simulink model "пример"  (R2023a)
settings: Solver=VariableStepAuto  StartTime=0.0  StopTime=10.0  RelTol=1e-3
libraries: simulink x1
settings Model: Creator=artemii  LastModifiedBy=Theomur

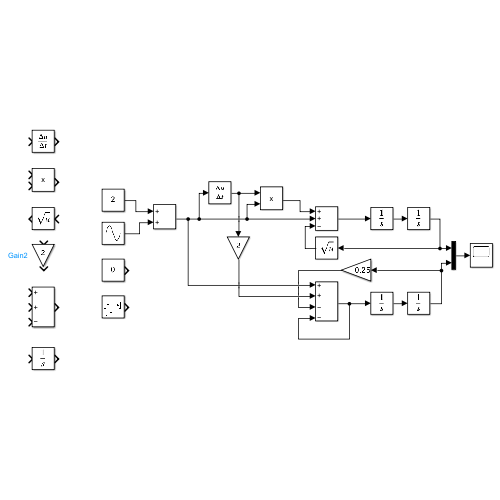
[thumbnail: Simulink's stored preview of the top-level diagram]
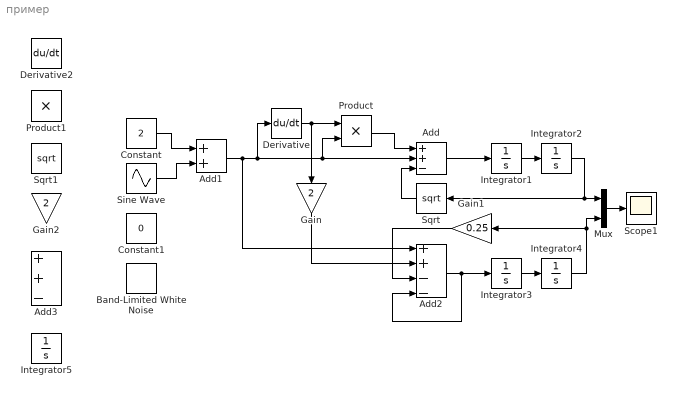
== system пример ==
  Add : Sum  Inputs=++-
  Add1 : Sum
  Add2 : Sum  Inputs=++--
  Add3 : Sum  Inputs=++-
  Band-Limited White Noise : simulink/Sources/Band-Limited White Noise  Cov=[0.1]  Ts=0.1  seed=[12345]
  Constant : Constant  Value=2
  Constant1 : Constant  Value=0
  Derivative : Derivative
  Derivative2 : Derivative
  Gain : Gain  Gain=2
  Gain1 : Gain  Gain=0.25
  Gain2 : Gain  Gain=2
  Integrator{1..5} (5 alike) : Integrator
  Mux : Mux  Inputs=2
  Product : Product
  Product1 : Product
  Scope1 : Scope
  Sine Wave : Sin  SampleTime=0
  Sqrt : Sqrt
  Sqrt1 : Sqrt
  wires:
  Constant/1 -> Add1/1
  Integrator1/1 -> Integrator2/1
  Sqrt/1 -> Add/3
  Product/1 -> Add/1
  Add1/1 -> Add2/1, Derivative/1, Product/2, Add/2
  Derivative/1 -> Gain/1, Product/1
  Add/1 -> Integrator1/1
  Integrator2/1 -> Sqrt/1, Mux/1
  Mux/1 -> Scope1/1
  Gain/1 -> Add2/2
  Gain1/1 -> Add2/3
  Integrator3/1 -> Integrator4/1
  Add2/1 -> Add2/4, Integrator3/1
  Integrator4/1 -> Mux/2, Gain1/1
  Sine Wave/1 -> Add1/2
